simulink model "Three_phase_halfwave_rectifier"  (R2025b)
settings: Solver=ode23tb  StartTime=0.0  StopTime=0.1  RelTol=1e-3
libraries: spsACVoltageSourceLib x9, spsDiodeLib x6, spsGroundLib x6, spsCurrentMeasurementLib x3, spsSeriesRLCBranchLib x3, spsThreePhaseVIMeasurementLib x3, spsThyristorLib x3, spsVoltageMeasurementLib x3, sps_lib x1
settings Model: Creator=Luqmaan  LastModifiedBy=Luqmaan

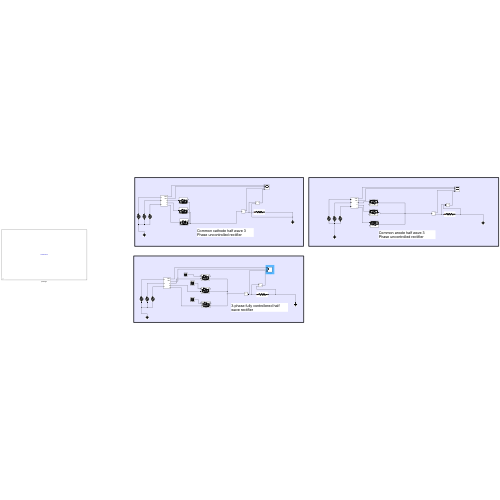
[thumbnail: Simulink's stored preview of the top-level diagram]
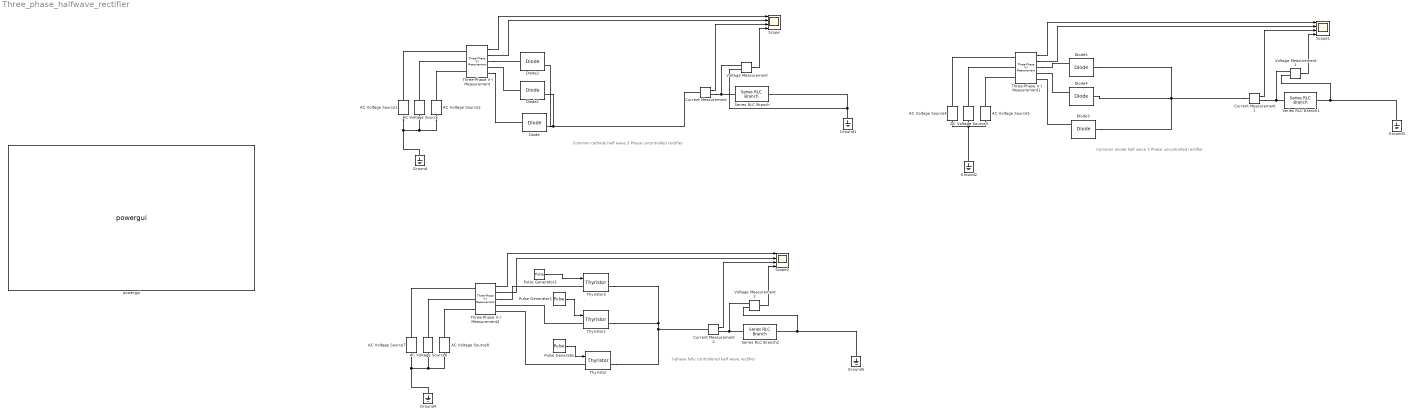
== system Three_phase_halfwave_rectifier ==
  note: 3-phase fully controllered half wave rectifier
  note: Common anode half wave 3 Phase uncontrolled rectifier
  note: Common cathode half wave 3 Phase uncontrolled rectifier
  AC Voltage Source : spsACVoltageSourceLib/AC Voltage Source  Amplitude=400  Phase=0  Frequency=50  SampleTime=0  Measurements=None  BusType=swing  Pref=10e3  Qref=0  Qmin=-inf  Qmax=+inf
  AC Voltage Source1 : spsACVoltageSourceLib/AC Voltage Source  Amplitude=400  Phase=-120  Frequency=50  SampleTime=0  Measurements=None  BusType=swing  Pref=10e3  Qref=0  Qmin=-inf  Qmax=+inf
  AC Voltage Source2 : spsACVoltageSourceLib/AC Voltage Source  Amplitude=400  Phase=120  Frequency=50  SampleTime=0  Measurements=None  BusType=swing  Pref=10e3  Qref=0  Qmin=-inf  Qmax=+inf
  AC Voltage Source3 : spsACVoltageSourceLib/AC Voltage Source  Amplitude=400  Phase=0  Frequency=50  SampleTime=0  Measurements=None  BusType=swing  Pref=10e3  Qref=0  Qmin=-inf  Qmax=+inf
  AC Voltage Source4 : spsACVoltageSourceLib/AC Voltage Source  Amplitude=400  Phase=-120  Frequency=50  SampleTime=0  Measurements=None  BusType=swing  Pref=10e3  Qref=0  Qmin=-inf  Qmax=+inf
  AC Voltage Source5 : spsACVoltageSourceLib/AC Voltage Source  Amplitude=400  Phase=120  Frequency=50  SampleTime=0  Measurements=None  BusType=swing  Pref=10e3  Qref=0  Qmin=-inf  Qmax=+inf
  AC Voltage Source6 : spsACVoltageSourceLib/AC Voltage Source  Amplitude=400  Phase=120  Frequency=50  SampleTime=0  Measurements=None  BusType=swing  Pref=10e3  Qref=0  Qmin=-inf  Qmax=+inf
  AC Voltage Source7 : spsACVoltageSourceLib/AC Voltage Source  Amplitude=400  Phase=0  Frequency=50  SampleTime=0  Measurements=None  BusType=swing  Pref=10e3  Qref=0  Qmin=-inf  Qmax=+inf
  AC Voltage Source8 : spsACVoltageSourceLib/AC Voltage Source  Amplitude=400  Phase=240  Frequency=50  SampleTime=0  Measurements=None  BusType=swing  Pref=10e3  Qref=0  Qmin=-inf  Qmax=+inf
  Current Measurement : spsCurrentMeasurementLib/Current Measurement  PhasorSimulation=off  OutputType=Complex  PSBequivalent=0
  Current Measurement1 : spsCurrentMeasurementLib/Current Measurement  PhasorSimulation=off  OutputType=Complex  PSBequivalent=0
  Current Measurement2 : spsCurrentMeasurementLib/Current Measurement  PhasorSimulation=off  OutputType=Complex  PSBequivalent=0
  Diode{,1..5} (6 alike) : spsDiodeLib/Diode  Ron=0.001  Lon=0  Vf=0.8  IC=0  UseSnubber=0  Rs=500  Cs=250e-9  Measurements=on
  Ground{,1..5} (6 alike) : spsGroundLib/Ground  LConnTagsString=a
  Pulse Generator : DiscretePulseGenerator  PulseType=Time based  Period=0.02  PulseWidth=5  PhaseDelay=(0.02/360)*300
  Pulse Generator1 : DiscretePulseGenerator  PulseType=Time based  Period=0.02  PulseWidth=5  PhaseDelay=(0.02/360)*180
  Pulse Generator2 : DiscretePulseGenerator  PulseType=Time based  Period=0.02  PulseWidth=5  PhaseDelay=(0.02/360)*60
  Scope : Scope  NumInputPorts=4
      settings: ActiveDisplayYMinimum=-499.9964026926433  ActiveDisplayYMaximum=499.967624249017
  Scope1 : Scope  NumInputPorts=4
      settings: ActiveDisplayYMinimum=-499.99999999809546  ActiveDisplayYMaximum=499.99999999809614
  Scope2 : Scope  NumInputPorts=4
      settings: ActiveDisplayYMinimum=-499.9999999980966  ActiveDisplayYMaximum=499.999999998096  DataLoggingVariableName=ScopeData2
  Series RLC Branch : spsSeriesRLCBranchLib/Series RLC Branch  LConnTagsString=__new0  RConnTagsString=__new0  BranchType=R  Resistance=100  Inductance=1e-3  SetiL0=off  InitialCurrent=0  Capacitance=1e-6  Setx0=off  InitialVoltage=0  Measurements=None
  Series RLC Branch1 : spsSeriesRLCBranchLib/Series RLC Branch  LConnTagsString=__new0  RConnTagsString=__new0  BranchType=R  Resistance=100  Inductance=1e-3  SetiL0=off  InitialCurrent=0  Capacitance=1e-6  Setx0=off  InitialVoltage=0  Measurements=None
  Series RLC Branch2 : spsSeriesRLCBranchLib/Series RLC Branch  LConnTagsString=__new0  RConnTagsString=__new0  BranchType=R  Resistance=100  Inductance=1e-3  SetiL0=off  InitialCurrent=0  Capacitance=1e-6  Setx0=off  InitialVoltage=0  Measurements=None
  Three-Phase V-I Measurement : spsThreePhaseVIMeasurementLib/Three-Phase V-I Measurement  VoltageMeasurement=phase-to-ground  SetLabelV=off  LabelV=Vabc  Vpu=off  VpuLL=off  CurrentMeasurement=yes  SetLabelI=off  LabelI=Iabc  Ipu=off  Pbase=100e6  Vbase=500e3  OutputType=Complex  PhasorSimulation=off  PSBequivalent=0
  Three-Phase V-I Measurement1 : spsThreePhaseVIMeasurementLib/Three-Phase V-I Measurement  VoltageMeasurement=phase-to-ground  SetLabelV=off  LabelV=Vabc  Vpu=off  VpuLL=off  CurrentMeasurement=yes  SetLabelI=off  LabelI=Iabc  Ipu=off  Pbase=100e6  Vbase=500e3  OutputType=Complex  PhasorSimulation=off  PSBequivalent=0
  Three-Phase V-I Measurement2 : spsThreePhaseVIMeasurementLib/Three-Phase V-I Measurement  VoltageMeasurement=phase-to-ground  SetLabelV=off  LabelV=Vabc  Vpu=off  VpuLL=off  CurrentMeasurement=yes  SetLabelI=off  LabelI=Iabc  Ipu=off  Pbase=100e6  Vbase=500e3  OutputType=Complex  PhasorSimulation=off  PSBequivalent=0
  Thyristor : spsThyristorLib/Thyristor  Ron=0.001  Lon=0  Vf=0.8  IC=0  Rs=500  Cs=250e-9  Measurements=on
  Thyristor1 : spsThyristorLib/Thyristor  Ron=0.001  Lon=0  Vf=0.8  IC=0  Rs=500  Cs=250e-9  Measurements=on
  Thyristor2 : spsThyristorLib/Thyristor  Ron=0.001  Lon=0  Vf=0.8  IC=0  Rs=500  Cs=250e-9  Measurements=on
  Voltage Measurement : spsVoltageMeasurementLib/Voltage Measurement  PhasorSimulation=off  OutputType=Complex  PSBequivalent=0
  Voltage Measurement1 : spsVoltageMeasurementLib/Voltage Measurement  PhasorSimulation=off  OutputType=Complex  PSBequivalent=0
  Voltage Measurement2 : spsVoltageMeasurementLib/Voltage Measurement  PhasorSimulation=off  OutputType=Complex  PSBequivalent=0
  powergui : sps_lib/powergui  Priority=1  SimulationMode=Continuous  SampleTime=50e-6  frequency=60  Iterations=50  frequencyindice=50  Pbase=100e6  ErrMax=1e-4  UnitsV=kV  UnitsW=MW  buscounter=0  FunctionMessages=off  echomessages=off  EnableUseOfTLC=off  CurrentSourceSwitches=off  DisableSnubberDevices=off  DisableRonSwitches=off  DisableVfSwitches=off  DisplayEquations=off  AutomaticDiscreteSolvers=off  SolverType=Tustin/Backward Euler (TBE)  Interpol=off  ExternalGateDelay=off  methode=off  Ts=100  x0status=blocks  SPID=on  SwTol=0  HookPort=off  NonlinearTolerance=1e-4  nMaxIteration=100  ContinueOnMaxIteration=off  RestoreLinks=warning  ResistiveCurrentMeasurement=off  Frange=[0:2:500]  Ylog=off  Xlog=on  ShowGrid=off  save=off  variable=ZData  structure=0  ZoomFFT=off  StartTime=0.0  cycles=1  DisplayStyle=1  fundamental=60  FreqAxis=off  MaxFrequency=1000  frequencyindicesteady=1  RmsSteady=1  display=off
  wires:
  Current Measurement1/1 -> Scope1/3
  Voltage Measurement1/1 -> Scope1/4
  Three-Phase V-I Measurement1/2 -> Scope1/2
  Three-Phase V-I Measurement1/1 -> Scope1/1
  Voltage Measurement/1 -> Scope/4
  Current Measurement/1 -> Scope/3
  Three-Phase V-I Measurement/1 -> Scope/1
  Three-Phase V-I Measurement/2 -> Scope/2
  Voltage Measurement2/1 -> Scope2/4
  Current Measurement2/1 -> Scope2/3
  Three-Phase V-I Measurement2/1 -> Scope2/1
  Three-Phase V-I Measurement2/2 -> Scope2/2
  Pulse Generator2/1 -> Thyristor2/1
  Pulse Generator1/1 -> Thyristor1/1
  Pulse Generator/1 -> Thyristor/1
  connections:
  Current Measurement1/LConn1 -- Diode5/LConn1 -- Diode4/LConn1 -- Diode3/LConn1
  Current Measurement1/RConn1 -- Voltage Measurement1/LConn1 -- Series RLC Branch1/LConn1
  AC Voltage Source4/LConn1 -- AC Voltage Source5/LConn1 -- Ground2/LConn1 -- AC Voltage Source3/LConn1
  Series RLC Branch1/RConn1 -- Ground3/LConn1 -- Voltage Measurement1/LConn2
  Diode3/RConn1 -- Three-Phase V-I Measurement1/RConn3
  AC Voltage Source4/RConn1 -- Three-Phase V-I Measurement1/LConn1
  AC Voltage Source5/RConn1 -- Three-Phase V-I Measurement1/LConn3
  AC Voltage Source3/RConn1 -- Three-Phase V-I Measurement1/LConn2
  Diode4/RConn1 -- Three-Phase V-I Measurement1/RConn2
  Three-Phase V-I Measurement1/RConn1 -- Diode5/RConn1
  Series RLC Branch/RConn1 -- Ground1/LConn1 -- Voltage Measurement/LConn2
  AC Voltage Source/LConn1 -- AC Voltage Source1/LConn1 -- Ground/LConn1 -- AC Voltage Source2/LConn1
  Current Measurement/RConn1 -- Series RLC Branch/LConn1 -- Voltage Measurement/LConn1
  Diode1/RConn1 -- Current Measurement/LConn1 -- Diode2/RConn1 -- Diode/RConn1
  Three-Phase V-I Measurement/RConn1 -- Diode2/LConn1
  Diode1/LConn1 -- Three-Phase V-I Measurement/RConn2
  Three-Phase V-I Measurement/RConn3 -- Diode/LConn1
  AC Voltage Source2/RConn1 -- Three-Phase V-I Measurement/LConn3
  AC Voltage Source/RConn1 -- Three-Phase V-I Measurement/LConn2
  AC Voltage Source1/RConn1 -- Three-Phase V-I Measurement/LConn1
  Series RLC Branch2/RConn1 -- Ground5/LConn1 -- Voltage Measurement2/LConn2
  AC Voltage Source6/LConn1 -- AC Voltage Source7/LConn1 -- Ground4/LConn1 -- AC Voltage Source8/LConn1
  Current Measurement2/RConn1 -- Series RLC Branch2/LConn1 -- Voltage Measurement2/LConn1
  AC Voltage Source6/RConn1 -- Three-Phase V-I Measurement2/LConn2
  AC Voltage Source7/RConn1 -- Three-Phase V-I Measurement2/LConn1
  AC Voltage Source8/RConn1 -- Three-Phase V-I Measurement2/LConn3
  Three-Phase V-I Measurement2/RConn1 -- Thyristor2/LConn1
  Thyristor1/LConn1 -- Three-Phase V-I Measurement2/RConn2
  Thyristor/LConn1 -- Three-Phase V-I Measurement2/RConn3
  Thyristor2/RConn1 -- Current Measurement2/LConn1 -- Thyristor/RConn1 -- Thyristor1/RConn1
